simulink model "MyOwnProject"  (R2025a)
settings: Solver=ode23s  StartTime=0.0  StopTime=50  MaxStep=0.2  RelTol=1e-3
settings Model: Creator=sanghoon  LastModifiedBy=sanghoon

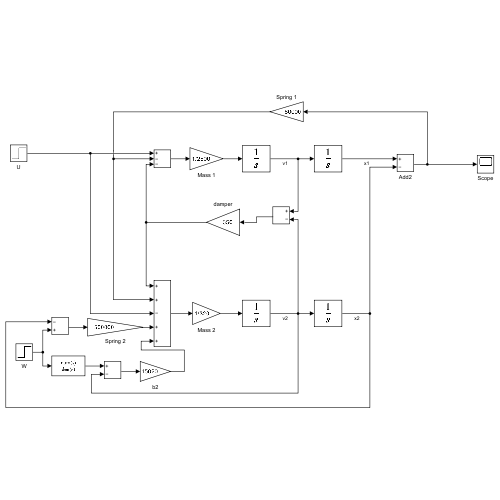
[thumbnail: Simulink's stored preview of the top-level diagram]
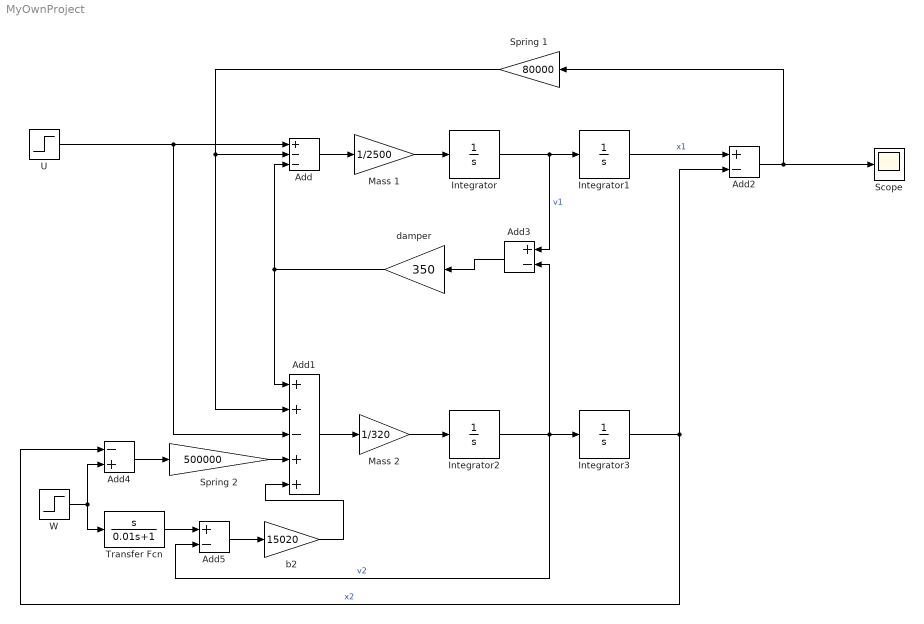
== system MyOwnProject ==
  Add : Sum  Inputs=+--
  Add1 : Sum  Inputs=++-++
  Add2 : Sum  Inputs=+-
  Add3 : Sum  Inputs=+-
  Add4 : Sum  Inputs=-+
  Add5 : Sum  Inputs=+-
  Integrator{,1..3} (4 alike) : Integrator
  Mass 1 : Gain  Gain=1/2500
  Mass 2 : Gain  Gain=1/320
  Scope : Scope
      settings: ActiveDisplayYMinimum=-0.413879766423324  ActiveDisplayYMaximum=0.53555892712977982
  Spring 1 : Gain  Gain=80000
  Spring 2 : Gain  Gain=500000
  Transfer Fcn : TransferFcn  Numerator=[1 0]  Denominator=[0.01 1]
  U : Step  Time=0  SampleTime=0
  W : Step  After=0.1  SampleTime=0
  b2 : Gain  Gain=15020
  damper : Gain  Gain=350
  wires:
  Integrator/1 -> Add3/1, Integrator1/1  "v1"
  Integrator2/1 -> Add5/2, Add3/2, Integrator3/1  "v2"
  Mass 1/1 -> Integrator/1
  Mass 2/1 -> Integrator2/1
  Add/1 -> Mass 1/1
  Add1/1 -> Mass 2/1
  Integrator1/1 -> Add2/1  "x1"
  Integrator3/1 -> Add2/2, Add4/1  "x2"
  Add2/1 -> Spring 1/1, Scope/1
  Spring 1/1 -> Add/2, Add1/2
  Add3/1 -> damper/1
  damper/1 -> Add/3, Add1/1
  Spring 2/1 -> Add1/4
  Add4/1 -> Spring 2/1
  W/1 -> Transfer Fcn/1, Add4/2
  Add5/1 -> b2/1
  b2/1 -> Add1/5
  U/1 -> Add/1, Add1/3
  Transfer Fcn/1 -> Add5/1
